simulink model "hopsim3model"  (R2023b)
settings: Solver=VariableStepAuto  StartTime=0.0  StopTime=10.0  RelTol=1e-3
libraries: shared6dof x1
settings Model: Creator=jacksonwright  LastModifiedBy=jacksonwright

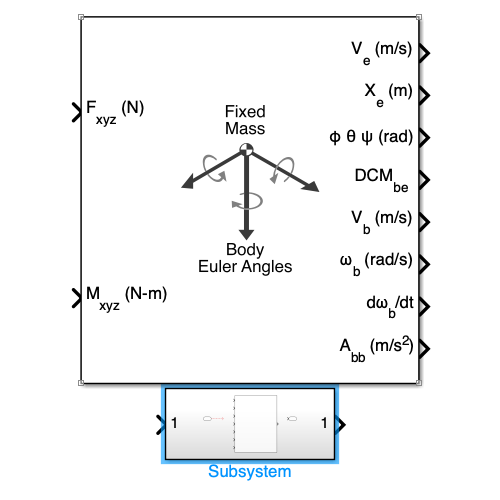
[thumbnail: Simulink's stored preview of the top-level diagram]
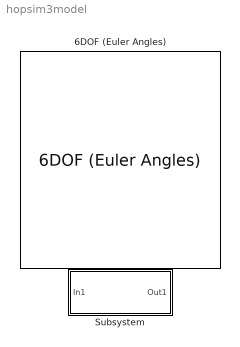
== system hopsim3model ==
  6DOF (Euler Angles) : shared6dof/6DOF (Euler Angles)  units=Metric (MKS)  mtype=Fixed  rep=Euler Angles  xme_0=[0 0 0]  Vm_0=[0 0 0]  eul_0=[0 0 0]  pm_0=[0 0 0]  mass_0=1.0  mass_e=0.5  mass_f=2.0  inertia=eye(3)  inertia_e=eye(3)  inertia_f=2*eye(3)  k_quat=1.0  vre_flag=on  abi_flag=off  aMode=0  xme_statename=''  Vm_statename=''  eul_statename=''  quat_statename=''  pm_statename=''  mass_statename=''
  Subsystem : Subsystem

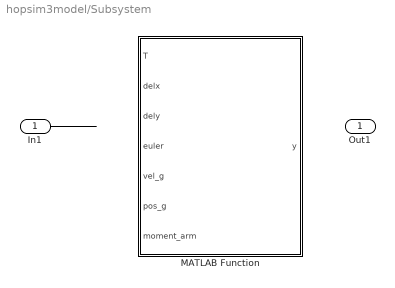
== system hopsim3model/Subsystem ==
  In1 : Inport
  MATLAB Function : MATLAB Function  TreatAsAtomicUnit=on
  Out1 : Outport
  wires:
  In1/1 -> ?

== matlab function hopsim3model/Subsystem/MATLAB Function ==
  data: T input; y output; delx input; dely input; euler input; vel_g input; pos_g input; moment_arm input
function y = fcn(T,delx,dely,euler,vel_g,pos_g, moment_arm)


force_thrust_b = T*[sin(dely)*cos(delx); -sin(delx); cos(dely)*cos(delx)]

tau = moment_arm * force_thrust;




y = u;
